simulink model "cl2"  (R2019b)
settings: Solver=VariableStepAuto  StartTime=0.0  StopTime=10.0  RelTol=1e-3
undefined symbols (not defined in the file or in its folder): A_cl, B_cl, C_cl, D_cl, K
settings Model: Creator=elina  LastModifiedBy=elina

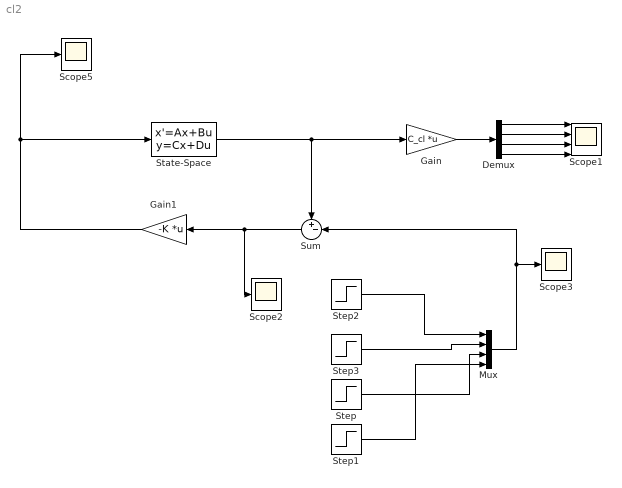
== system cl2 ==
  Demux : Demux
  Gain : Gain  Gain=C_cl  Multiplication=Matrix(K*u)
  Gain1 : Gain  Gain=-K  Multiplication=Matrix(K*u)
  Mux : Mux
  Scope1 : Scope  NumInputPorts=4
  Scope2 : Scope
  Scope3 : Scope
  Scope5 : Scope
  State-Space : StateSpace  A=A_cl  B=B_cl  C=C_cl  D=D_cl  InitialCondition=[0 2.8 0 0]
  Step : Step  Time=0  After=0  SampleTime=0
  Step1 : Step  After=0  SampleTime=0
  Step2 : Step  Time=0  After=10  SampleTime=0
  Step3 : Step  After=0  SampleTime=0
  Sum : Sum  Inputs=+-|
  wires:
  Gain/1 -> Demux/1
  Demux/1 -> Scope1/1
  Demux/2 -> Scope1/2
  Demux/3 -> Scope1/3
  Demux/4 -> Scope1/4
  Gain1/1 -> Scope5/1, State-Space/1
  State-Space/1 -> Sum/1, Gain/1
  Sum/1 -> Gain1/1, Scope2/1
  Step2/1 -> Mux/1
  Step3/1 -> Mux/2
  Step/1 -> Mux/3
  Step1/1 -> Mux/4
  Mux/1 -> Sum/2, Scope3/1
